simulink model "CryoDetXray"  (R2016b)
settings: Solver=ode45  StartTime=0.0  StopTime=10e-5  MaxStep=Tclk/4  RelTol=1e-3
values from neighbouring files (symbols this model uses):
  Fclk = Fadc    (= 307200000)    [setupCryoFPGAxray.m]
  Tclk = 1/Fclk    (= 3.25520833333e-09)    [setupCryoFPGAxray.m]
undefined symbols (not defined in the file or in its folder): AXI4, Lite, lpf, Naxi, xlipgetpartsetting
libraries: xbsIndex_r4 x1091, CryoDetLib x68, simulink x4, hdlsllib x1
(part 3 of 8)

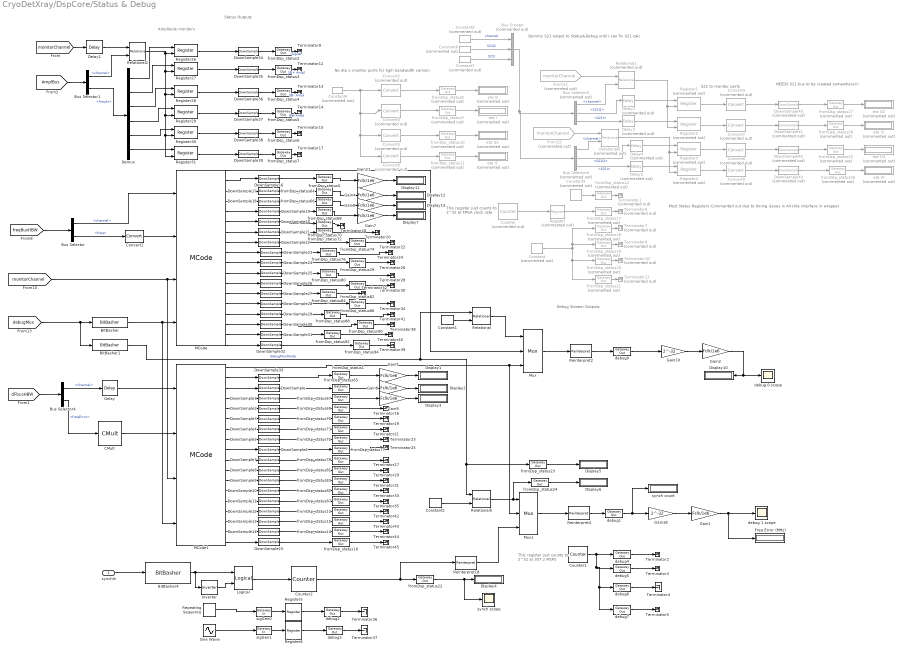
== system CryoDetXray/DspCore/Status & Debug ==
  note: Most Status Registers Commented out due to timing issues in AXI-lite interface in wrapper
  note: Dummy S21 output to Status&Debug until I can fix S21 calc
  note: No eta o monitor ports for hgih bandwidth version
  note: NEEDS S21 bus to be created somewhere!!!
  note: Amplitude monitors
  note: This register just counts to 2^32 at FPGA clock rate
  note: Status Outputs
  note: Debug Stream Outputs
  note: S21 to monitor ports
  note: This register just counts to 2^32 at 307.2 MSPS
  synchIn : Inport
  BitBasher : xbsIndex_r4/BitBasher  bitexpr=a={b[4:0]}  display_expr=on  sr_1=a  arith_type1=Unsigned  bin_pt1=0  sr_2=2  arith_type2=Unsigned  bin_pt2=0  sr_3=3  arith_type3=Unsigned  bin_pt3=0  sr_4=4  arith_type4=Unsigned  bin_pt4=0  dbl_ovrd=off  block_type=bitbasher
  BitBasher1 : xbsIndex_r4/BitBasher  bitexpr=a={b[6:5]}  display_expr=on  sr_1=a  arith_type1=Unsigned  bin_pt1=0  sr_2=2  arith_type2=Unsigned  bin_pt2=0  sr_3=3  arith_type3=Unsigned  bin_pt3=0  sr_4=4  arith_type4=Unsigned  bin_pt4=0  dbl_ovrd=off  block_type=bitbasher
  BitBasher4 : xbsIndex_r4/BitBasher  bitexpr=trig={Din[0]}  display_expr=on  sr_1=trig  arith_type1=Unsigned  bin_pt1=0  sr_2=2  arith_type2=Unsigned  bin_pt2=0  sr_3=3  arith_type3=Unsigned  bin_pt3=0  sr_4=4  arith_type4=Unsigned  bin_pt4=0  dbl_ovrd=off  block_type=bitbasher
  Bus Creator : BusCreator  Commented=on  Inputs=3
  Bus Selector : BusSelector  OutputSignals=channel,freq
  Bus Selector1 : BusSelector  OutputSignals=channel,Ampls
  Bus Selector4 : BusSelector  OutputSignals=channel,freqError
  Bus Selector5 : BusSelector  Commented=on  OutputSignals=channel,S21Q,S21I
  Bus Selector6 : BusSelector  Commented=on  OutputSignals=channel,S21Q,S21I
  CMult : xbsIndex_r4/CMult  const=16  gui_display_data_type=Fixed-point  const_n_bits=5  const_bin_pt=0  float_type=Single  exp_bits=8  fraction_bits=24  en=off  latency=3  precision=User Defined  arith_type="Signed  (2's comp)"  n_bits=32  bin_pt=31  quantization=Truncate  overflow=Saturate  use_behavioral_HDL=off  mem_type=Distributed RAM  pipeline=off  dbl_ovrd=off  block_type=cmult
  Constant : xbsIndex_r4/Constant  Commented=on  const=1.0  gui_display_data_type=Fixed-point  arith_type=Signed (2's comp)  n_bits=32  bin_pt=0  preci_type=Single  exp_width=8  frac_width=24  explicit_period=on  period=Tclk*Naxi  equ=P=C  opselect=C  inp2=PCIN>>17  opr=+  inp1=P  carry=CIN  dbl_ovrd=off  block_type=constant
  Constant1 : xbsIndex_r4/Constant  const=1  gui_display_data_type=Fixed-point  arith_type=Unsigned  n_bits=4  bin_pt=0  preci_type=Single  exp_width=8  frac_width=24  explicit_period=off  period=1  equ=P=C  opselect=C  inp2=PCIN>>17  opr=+  inp1=P  carry=CIN  dbl_ovrd=off  block_type=constant
  Constant2 : xbsIndex_r4/Constant  const=0  gui_display_data_type=Fixed-point  arith_type=Unsigned  n_bits=4  bin_pt=0  preci_type=Single  exp_width=8  frac_width=24  explicit_period=off  period=1  equ=P=C  opselect=C  inp2=PCIN>>17  opr=+  inp1=P  carry=CIN  dbl_ovrd=off  block_type=constant
  Constant3 : xbsIndex_r4/Constant  Commented=on  const=0  gui_display_data_type=Fixed-point  arith_type=Unsigned  n_bits=32  bin_pt=0  preci_type=Single  exp_width=8  frac_width=24  explicit_period=on  period=Tclk*Naxi  equ=P=C  opselect=C  inp2=PCIN>>17  opr=+  inp1=P  carry=CIN  dbl_ovrd=off  block_type=constant
  Constant4 : xbsIndex_r4/Constant  Commented=on  const=0  gui_display_data_type=Fixed-point  arith_type=Signed (2's comp)  n_bits=16  bin_pt=14  preci_type=Single  exp_width=8  frac_width=24  explicit_period=on  period=Tclk*Naxi  equ=P=C  opselect=C  inp2=PCIN>>17  opr=+  inp1=P  carry=CIN  dbl_ovrd=off  block_type=constant
  Constant5 : xbsIndex_r4/Constant  Commented=on  const=0  gui_display_data_type=Fixed-point  arith_type=Unsigned  n_bits=4  bin_pt=4  preci_type=Single  exp_width=8  frac_width=24  explicit_period=on  period=Tclk  equ=P=C  opselect=C  inp2=PCIN>>17  opr=+  inp1=P  carry=CIN  dbl_ovrd=off  block_type=constant
  Constant6 : xbsIndex_r4/Constant  Commented=on  const=0  gui_display_data_type=Fixed-point  arith_type=Signed (2's comp)  n_bits=32  bin_pt=14  preci_type=Single  exp_width=8  frac_width=24  explicit_period=on  period=Tclk  equ=P=C  opselect=C  inp2=PCIN>>17  opr=+  inp1=P  carry=CIN  dbl_ovrd=off  block_type=constant
  Constant7 : xbsIndex_r4/Constant  Commented=on  const=0  gui_display_data_type=Fixed-point  arith_type=Signed (2's comp)  n_bits=16  bin_pt=14  preci_type=Single  exp_width=8  frac_width=24  explicit_period=on  period=Tclk  equ=P=C  opselect=C  inp2=PCIN>>17  opr=+  inp1=P  carry=CIN  dbl_ovrd=off  block_type=constant
  Convert1 : xbsIndex_r4/Convert  gui_display_data_type=Fixed-point  arith_type="Signed  (2's comp)"  n_bits=32  bin_pt=31  float_type=Single  exp_bits=8  fraction_bits=24  quantization=Truncate  overflow=Wrap  en=off  latency=0  pipeline=off  dbl_ovrd=off  block_type=convert
  Convert{2..3,5..6} (4 alike) : xbsIndex_r4/Convert  Commented=on  gui_display_data_type=Fixed-point  arith_type="Signed  (2's comp)"  n_bits=32  bin_pt=14  float_type=Single  exp_bits=8  fraction_bits=24  quantization="Round  (unbiased: +/- Inf)"  overflow=Saturate  en=off  latency=1  pipeline=off  dbl_ovrd=off  block_type=convert
  Convert{4,7..9} (4 alike) : xbsIndex_r4/Convert  Commented=on  gui_display_data_type=Fixed-point  arith_type="Signed  (2's comp)"  n_bits=32  bin_pt=14  float_type=Single  exp_bits=8  fraction_bits=24  quantization="Round  (unbiased: +/- Inf)"  overflow=Saturate  en=off  latency=2  pipeline=off  dbl_ovrd=off  block_type=convert
  Counter : xbsIndex_r4/Counter  Commented=on  cnt_type=Free Running  cnt_to=Inf  operation=Up  start_count=0  cnt_by_val=1  arith_type=Unsigned  n_bits=32  bin_pt=0  load_pin=off  rst=off  en=off  explicit_period=on  period=Tclk*Naxi  use_behavioral_HDL=off  implementation=Fabric  dbl_ovrd=off  block_type=counter
  Counter1 : xbsIndex_r4/Counter  cnt_type=Free Running  cnt_to=Inf  operation=Up  start_count=0  cnt_by_val=1  arith_type=Unsigned  n_bits=32  bin_pt=0  load_pin=off  rst=off  en=off  explicit_period=on  period=Tclk  use_behavioral_HDL=off  implementation=Fabric  dbl_ovrd=off  block_type=counter
  Counter2 : xbsIndex_r4/Counter  cnt_type=Free Running  cnt_to=Inf  operation=Up  start_count=0  cnt_by_val=1  arith_type=Unsigned  n_bits=32  bin_pt=0  load_pin=off  rst=on  en=off  explicit_period=off  period=1  use_behavioral_HDL=on  implementation=Fabric  dbl_ovrd=off  block_type=counter
  Delay : xbsIndex_r4/Delay  rst=off  infoeditControl=Selection of Reset will increase slice count due to use of real FFs and instead of SRLs  en=off  latency=3  reg_retiming=off  dbl_ovrd=off  block_type=delay
      settings: infoedit=Hardware notes: A delay line is a chain, each link of which is an SRL16 or SRL32 followed by a flip-flop.
  Delay1 : xbsIndex_r4/Delay  rst=off  infoeditControl=Selection of Reset will increase slice count due to use of real FFs and instead of SRLs  en=off  latency=1  reg_retiming=on  dbl_ovrd=off  block_type=delay
  Delay{2..5} (4 alike) : xbsIndex_r4/Delay  Commented=on  rst=off  infoeditControl=Selection of Reset will increase slice count due to use of real FFs and instead of SRLs  en=off  latency=1  reg_retiming=on  dbl_ovrd=off  block_type=delay
  Demux : Demux  Outputs=6
  Display{1..7,10..13} (11 alike) : Display
      Display1 settings: Decimation=144
      Display10 settings: Decimation=144
      Display11 settings: Decimation=144
      Display12 settings: Decimation=144
      Display13 settings: Decimation=144
      Display2 settings: Decimation=144
      Display3 settings: Decimation=144
      Display7 settings: Decimation=144
  DownSample{,1..39} (40 alike) : CryoDetLib/DownSample
  DownSample{40..43} (4 alike) : CryoDetLib/DownSample  Commented=on
  Freq Error (MHz) : Display
      settings: Decimation=144
  From12 : From  Commented=on  GotoTag=monitorChannel  TagVisibility=global
  From15 : From  Commented=on  GotoTag=monitorChannel  TagVisibility=global
  Gain{1..2,4..9,21} (9 alike) : Gain  Gain=Fclk/1e6
  Gain10 : Gain  Gain=2^-32
  Gain18 : Gain  Gain=2^-32
  Inverter : xbsIndex_r4/Inverter  en=off  latency=1  dbl_ovrd=off  block_type=inv
  Logical : xbsIndex_r4/Logical  logical_function=AND  inputs=2  en=off  latency=1  precision=User Defined  arith_type=Boolean  n_bits=1  bin_pt=0  align_bp=on  dbl_ovrd=off  block_type=logical
  MCode : xbsIndex_r4/MCode  mfname=statusAndDebugPortsXray  explicit_period=off  period=1  inputsTable={'boundInpExpr'=>['','','',''],'inputs'=>['Chan','f','statusMux','debugMux']}  outputsTable={'outputs'=>['debugStream','fmon','f0','f1','f2','f3','f4','f5','f6','f7','f8','f9','f10','f11','f12','f13','f14','f15'],'suppressOut'=>['off','off','off','off','off','off','off','off','off','off','off','off','off','off','off','off','off','off']}  enable_stdout=off  enable_debug=off  suppress_output=on  defparams={}  hide_port_list={}  dbl_ovrd=off  block_type=mcode
  MCode1 : xbsIndex_r4/MCode  mfname=statusAndDebugPortsXray  explicit_period=off  period=1  inputsTable={'boundInpExpr'=>['','','',''],'inputs'=>['Chan','f','statusMux','debugMux']}  outputsTable={'outputs'=>['debugStream','fmon','f0','f1','f2','f3','f4','f5','f6','f7','f8','f9','f10','f11','f12','f13','f14','f15'],'suppressOut'=>['off','off','off','off','off','off','off','off','off','off','off','off','off','off','off','off','off','off']}  enable_stdout=off  enable_debug=on  suppress_output=on  defparams={}  hide_port_list={}  dbl_ovrd=off  block_type=mcode
  Mux : xbsIndex_r4/Mux  inputs=2  en=off  latency=0  precision=Full  arith_type=Unsigned  n_bits=16  bin_pt=14  quantization=Truncate  overflow=Wrap  dbl_ovrd=off  block_type=mux
  Mux1 : xbsIndex_r4/Mux  inputs=2  en=off  latency=0  precision=User Defined  arith_type="Signed  (2's comp)"  n_bits=32  bin_pt=31  quantization=Truncate  overflow=Saturate  dbl_ovrd=off  block_type=mux
  Register : xbsIndex_r4/Register  Commented=on  init=0  rst=off  en=off  dbl_ovrd=off  block_type=register
  Register{1..4} (4 alike) : xbsIndex_r4/Register  Commented=on  init=0  rst=off  en=on  dbl_ovrd=off  block_type=register
  Register{26..31} (6 alike) : xbsIndex_r4/Register  init=0  rst=off  en=on  dbl_ovrd=off  block_type=register
  Register5 : xbsIndex_r4/Register  init=1  rst=off  en=off  dbl_ovrd=off  block_type=register
  Register6 : xbsIndex_r4/Register  init=1  rst=off  en=off  dbl_ovrd=off  block_type=register
  Reinterpret18 : xbsIndex_r4/Reinterpret  force_arith_type=off  arith_type=Unsigned  force_bin_pt=on  bin_pt=32  block_type=reinterpret
  Reinterpret2 : xbsIndex_r4/Reinterpret  force_arith_type=on  arith_type=Unsigned  force_bin_pt=off  bin_pt=15  block_type=reinterpret
  Reinterpret4 : xbsIndex_r4/Reinterpret  force_arith_type=on  arith_type=Unsigned  force_bin_pt=off  bin_pt=15  block_type=reinterpret
  Relational : xbsIndex_r4/Relational  mode=a>b  op_type=Bool  en=off  latency=0  dbl_ovrd=off  block_type=relational
  Relational1 : xbsIndex_r4/Relational  Commented=on  mode=a=b  op_type=Bool  en=off  latency=1  dbl_ovrd=off  block_type=relational
  Relational2 : xbsIndex_r4/Relational  mode=a=b  op_type=Bool  en=off  latency=0  dbl_ovrd=off  block_type=relational
  Relational5 : xbsIndex_r4/Relational  mode=a!=b  op_type=Bool  en=off  latency=0  dbl_ovrd=off  block_type=relational
  Relational6 : xbsIndex_r4/Relational  Commented=on  mode=a=b  op_type=Bool  en=off  latency=1  dbl_ovrd=off  block_type=relational
  Repeating Sequence : simulink/Sources/Repeating Sequence  rep_seq_t="[0  2^32*Tclk]"  rep_seq_y=[0 1]
  Sine Wave : Sin  Amplitude=2^31  Bias=2^31  Frequency=2*pi*Fclk/2^32  SampleTime=0
  Terminator{1,6..8,10..11} (6 alike) : Terminator  Commented=on
  Terminator{2..5,9,12..45} (39 alike) : Terminator
  "debug 0 scope " : Scope
  debug 1 scope : Scope
  debug{0..7} (8 alike) : xbsIndex_r4/Gateway Out  inherit_from_input=on  hdl_port=on  rows=1  columns=1  UseAsDAC=off  DACChannel='1'  interface=None  automatic_assignment=on  address_offset=hex2dec('00')  intf_name=''  intf_description=''  timing_constraint=None  locs_specified=off  LOCs={}  io_standard={}  block_type=gatewayout
  eta I{,1..3} (4 alike) : Display  Commented=on
      settings: Decimation=144
  eta Q{,1..3} (4 alike) : Display  Commented=on
      settings: Decimation=144
  fromDsp_status0 : xbsIndex_r4/Gateway Out  inherit_from_input=on  hdl_port=on  rows=1  columns=1  UseAsDAC=off  DACChannel='1'  interface=AXI4-Lite  automatic_assignment=off  address_offset=hex2dec('00')  intf_name=''  intf_description=''  timing_constraint=None  locs_specified=off  LOCs={}  io_standard={}  block_type=gatewayout
  fromDsp_status1 : xbsIndex_r4/Gateway Out  inherit_from_input=on  hdl_port=on  rows=1  columns=1  UseAsDAC=off  DACChannel='1'  interface=AXI4-Lite  automatic_assignment=off  address_offset=hex2dec('04')  intf_name=''  intf_description=''  timing_constraint=None  locs_specified=off  LOCs={}  io_standard={}  block_type=gatewayout
  fromDsp_status10 : xbsIndex_r4/Gateway Out  Commented=on  inherit_from_input=on  hdl_port=on  rows=1  columns=1  UseAsDAC=off  DACChannel='1'  interface=AXI4-Lite  automatic_assignment=off  address_offset=hex2dec('28')  intf_name=''  intf_description=''  timing_constraint=None  locs_specified=off  LOCs={}  io_standard={}  block_type=gatewayout
  fromDsp_status11 : xbsIndex_r4/Gateway Out  Commented=on  inherit_from_input=on  hdl_port=on  rows=1  columns=1  UseAsDAC=off  DACChannel='1'  interface=AXI4-Lite  automatic_assignment=off  address_offset=hex2dec('2c')  intf_name=''  intf_description=''  timing_constraint=None  locs_specified=off  LOCs={}  io_standard={}  block_type=gatewayout
  fromDsp_status12 : xbsIndex_r4/Gateway Out  Commented=on  inherit_from_input=on  hdl_port=on  rows=1  columns=1  UseAsDAC=off  DACChannel='1'  interface=AXI4-Lite  automatic_assignment=off  address_offset=hex2dec('40')  intf_name=''  intf_description=''  timing_constraint=None  locs_specified=off  LOCs={}  io_standard={}  block_type=gatewayout
  fromDsp_status13 : xbsIndex_r4/Gateway Out  inherit_from_input=on  hdl_port=on  rows=1  columns=1  UseAsDAC=off  DACChannel='1'  interface=AXI4-Lite  automatic_assignment=off  address_offset=hex2dec('164')  intf_name=''  intf_description=''  timing_constraint=None  locs_specified=off  LOCs={}  io_standard={}  block_type=gatewayout
  fromDsp_status14 : xbsIndex_r4/Gateway Out  inherit_from_input=on  hdl_port=on  rows=1  columns=1  UseAsDAC=off  DACChannel='1'  interface=AXI4-Lite  automatic_assignment=off  address_offset=hex2dec('174')  intf_name=''  intf_description=''  timing_constraint=None  locs_specified=off  LOCs={}  io_standard={}  block_type=gatewayout
  fromDsp_status15 : xbsIndex_r4/Gateway Out  inherit_from_input=on  hdl_port=on  rows=1  columns=1  UseAsDAC=off  DACChannel='1'  interface=AXI4-Lite  automatic_assignment=off  address_offset=hex2dec('16c')  intf_name=''  intf_description=''  timing_constraint=None  locs_specified=off  LOCs={}  io_standard={}  block_type=gatewayout
  fromDsp_status16 : xbsIndex_r4/Gateway Out  inherit_from_input=on  hdl_port=on  rows=1  columns=1  UseAsDAC=off  DACChannel='1'  interface=AXI4-Lite  automatic_assignment=off  address_offset=hex2dec('17c')  intf_name=''  intf_description=''  timing_constraint=None  locs_specified=off  LOCs={}  io_standard={}  block_type=gatewayout
  fromDsp_status17 : xbsIndex_r4/Gateway Out  Commented=on  inherit_from_input=on  hdl_port=on  rows=1  columns=1  UseAsDAC=off  DACChannel='1'  interface=AXI4-Lite  automatic_assignment=off  address_offset=hex2dec('44')  intf_name=''  intf_description=''  timing_constraint=None  locs_specified=off  LOCs={}  io_standard={}  block_type=gatewayout
  fromDsp_status18 : xbsIndex_r4/Gateway Out  Commented=on  inherit_from_input=on  hdl_port=on  rows=1  columns=1  UseAsDAC=off  DACChannel='1'  interface=AXI4-Lite  automatic_assignment=off  address_offset=hex2dec('48')  intf_name=''  intf_description=''  timing_constraint=None  locs_specified=off  LOCs={}  io_standard={}  block_type=gatewayout
  fromDsp_status19 : xbsIndex_r4/Gateway Out  Commented=on  inherit_from_input=on  hdl_port=on  rows=1  columns=1  UseAsDAC=off  DACChannel='1'  interface=AXI4-Lite  automatic_assignment=off  address_offset=hex2dec('4c')  intf_name=''  intf_description=''  timing_constraint=None  locs_specified=off  LOCs={}  io_standard={}  block_type=gatewayout
  fromDsp_status2 : xbsIndex_r4/Gateway Out  inherit_from_input=on  hdl_port=on  rows=1  columns=1  UseAsDAC=off  DACChannel='1'  interface=AXI4-Lite  automatic_assignment=off  address_offset=hex2dec('08')  intf_name=''  intf_description=''  timing_constraint=None  locs_specified=off  LOCs={}  io_standard={}  block_type=gatewayout
  fromDsp_status20 : xbsIndex_r4/Gateway Out  Commented=on  inherit_from_input=on  hdl_port=on  rows=1  columns=1  UseAsDAC=off  DACChannel='1'  interface=AXI4-Lite  automatic_assignment=off  address_offset=hex2dec('50')  intf_name=''  intf_description=''  timing_constraint=None  locs_specified=off  LOCs={}  io_standard={}  block_type=gatewayout
  fromDsp_status21 : xbsIndex_r4/Gateway Out  Commented=on  inherit_from_input=on  hdl_port=on  rows=1  columns=1  UseAsDAC=off  DACChannel='1'  interface=AXI4-Lite  automatic_assignment=off  address_offset=hex2dec('54')  intf_name=''  intf_description=''  timing_constraint=None  locs_specified=off  LOCs={}  io_standard={}  block_type=gatewayout
  fromDsp_status22 : xbsIndex_r4/Gateway Out  inherit_from_input=on  hdl_port=off  rows=1  columns=1  UseAsDAC=off  DACChannel='1'  interface=AXI4-Lite  automatic_assignment=off  address_offset=hex2dec('30')  intf_name=''  intf_description=''  timing_constraint=None  locs_specified=off  LOCs={}  io_standard={}  block_type=gatewayout
  fromDsp_status23 : xbsIndex_r4/Gateway Out  inherit_from_input=on  hdl_port=off  rows=1  columns=1  UseAsDAC=off  DACChannel='1'  interface=AXI4-Lite  automatic_assignment=off  address_offset=hex2dec('30')  intf_name=''  intf_description=''  timing_constraint=None  locs_specified=off  LOCs={}  io_standard={}  block_type=gatewayout
  fromDsp_status24 : xbsIndex_r4/Gateway Out  inherit_from_input=on  hdl_port=off  rows=1  columns=1  UseAsDAC=off  DACChannel='1'  interface=AXI4-Lite  automatic_assignment=off  address_offset=hex2dec('30')  intf_name=''  intf_description=''  timing_constraint=None  locs_specified=off  LOCs={}  io_standard={}  block_type=gatewayout
  fromDsp_status25 : xbsIndex_r4/Gateway Out  Commented=on  inherit_from_input=on  hdl_port=on  rows=1  columns=1  UseAsDAC=off  DACChannel='1'  interface=AXI4-Lite  automatic_assignment=off  address_offset=hex2dec('38')  intf_name=''  intf_description=''  timing_constraint=None  locs_specified=off  LOCs={}  io_standard={}  block_type=gatewayout
  fromDsp_status26 : xbsIndex_r4/Gateway Out  Commented=on  inherit_from_input=on  hdl_port=on  rows=1  columns=1  UseAsDAC=off  DACChannel='1'  interface=AXI4-Lite  automatic_assignment=off  address_offset=hex2dec('3c')  intf_name=''  intf_description=''  timing_constraint=None  locs_specified=off  LOCs={}  io_standard={}  block_type=gatewayout
  fromDsp_status27 : xbsIndex_r4/Gateway Out  Commented=on  inherit_from_input=on  hdl_port=on  rows=1  columns=1  UseAsDAC=off  DACChannel='1'  interface=AXI4-Lite  automatic_assignment=off  address_offset=hex2dec('30')  intf_name=''  intf_description=''  timing_constraint=None  locs_specified=off  LOCs={}  io_standard={}  block_type=gatewayout
  fromDsp_status28 : xbsIndex_r4/Gateway Out  Commented=on  inherit_from_input=on  hdl_port=on  rows=1  columns=1  UseAsDAC=off  DACChannel='1'  interface=AXI4-Lite  automatic_assignment=off  address_offset=hex2dec('34')  intf_name=''  intf_description=''  timing_constraint=None  locs_specified=off  LOCs={}  io_standard={}  block_type=gatewayout
  fromDsp_status29 : xbsIndex_r4/Gateway Out  inherit_from_input=on  hdl_port=on  rows=1  columns=1  UseAsDAC=off  DACChannel='1'  interface=AXI4-Lite  automatic_assignment=off  address_offset=hex2dec('138')  intf_name=''  intf_description=''  timing_constraint=None  locs_specified=off  LOCs={}  io_standard={}  block_type=gatewayout
  fromDsp_status3 : xbsIndex_r4/Gateway Out  inherit_from_input=on  hdl_port=on  rows=1  columns=1  UseAsDAC=off  DACChannel='1'  interface=AXI4-Lite  automatic_assignment=off  address_offset=hex2dec('0C')  intf_name=''  intf_description=''  timing_constraint=None  locs_specified=off  LOCs={}  io_standard={}  block_type=gatewayout
  fromDsp_status4 : xbsIndex_r4/Gateway Out  inherit_from_input=on  hdl_port=on  rows=1  columns=1  UseAsDAC=off  DACChannel='1'  interface=AXI4-Lite  automatic_assignment=off  address_offset=hex2dec('10')  intf_name=''  intf_description=''  timing_constraint=None  locs_specified=off  LOCs={}  io_standard={}  block_type=gatewayout
  fromDsp_status5 : xbsIndex_r4/Gateway Out  inherit_from_input=on  hdl_port=on  rows=1  columns=1  UseAsDAC=off  DACChannel='1'  interface=AXI4-Lite  automatic_assignment=off  address_offset=hex2dec('14')  intf_name=''  intf_description=''  timing_constraint=None  locs_specified=off  LOCs={}  io_standard={}  block_type=gatewayout
  fromDsp_status6 : xbsIndex_r4/Gateway Out  inherit_from_input=on  hdl_port=on  rows=1  columns=1  UseAsDAC=off  DACChannel='1'  interface=AXI4-Lite  automatic_assignment=off  address_offset=hex2dec('18')  intf_name=''  intf_description=''  timing_constraint=None  locs_specified=off  LOCs={}  io_standard={}  block_type=gatewayout
  fromDsp_status64 : xbsIndex_r4/Gateway Out  inherit_from_input=on  hdl_port=on  rows=1  columns=1  UseAsDAC=off  DACChannel='1'  interface=AXI4-Lite  automatic_assignment=off  address_offset=hex2dec('100')  intf_name=''  intf_description=''  timing_constraint=None  locs_specified=off  LOCs={}  io_standard={}  block_type=gatewayout
  fromDsp_status65 : xbsIndex_r4/Gateway Out  inherit_from_input=on  hdl_port=on  rows=1  columns=1  UseAsDAC=off  DACChannel='1'  interface=AXI4-Lite  automatic_assignment=off  address_offset=hex2dec('104')  intf_name=''  intf_description=''  timing_constraint=None  locs_specified=off  LOCs={}  io_standard={}  block_type=gatewayout
  fromDsp_status66 : xbsIndex_r4/Gateway Out  inherit_from_input=on  hdl_port=on  rows=1  columns=1  UseAsDAC=off  DACChannel='1'  interface=AXI4-Lite  automatic_assignment=off  address_offset=hex2dec('108')  intf_name=''  intf_description=''  timing_constraint=None  locs_specified=off  LOCs={}  io_standard={}  block_type=gatewayout
  fromDsp_status67 : xbsIndex_r4/Gateway Out  inherit_from_input=on  hdl_port=on  rows=1  columns=1  UseAsDAC=off  DACChannel='1'  interface=AXI4-Lite  automatic_assignment=off  address_offset=hex2dec('10c')  intf_name=''  intf_description=''  timing_constraint=None  locs_specified=off  LOCs={}  io_standard={}  block_type=gatewayout
  fromDsp_status68 : xbsIndex_r4/Gateway Out  inherit_from_input=on  hdl_port=on  rows=1  columns=1  UseAsDAC=off  DACChannel='1'  interface=AXI4-Lite  automatic_assignment=off  address_offset=hex2dec('110')  intf_name=''  intf_description=''  timing_constraint=None  locs_specified=off  LOCs={}  io_standard={}  block_type=gatewayout
  fromDsp_status69 : xbsIndex_r4/Gateway Out  inherit_from_input=on  hdl_port=on  rows=1  columns=1  UseAsDAC=off  DACChannel='1'  interface=AXI4-Lite  automatic_assignment=off  address_offset=hex2dec('114')  intf_name=''  intf_description=''  timing_constraint=None  locs_specified=off  LOCs={}  io_standard={}  block_type=gatewayout
  fromDsp_status7 : xbsIndex_r4/Gateway Out  inherit_from_input=on  hdl_port=on  rows=1  columns=1  UseAsDAC=off  DACChannel='1'  interface=AXI4-Lite  automatic_assignment=off  address_offset=hex2dec('1C')  intf_name=''  intf_description=''  timing_constraint=None  locs_specified=off  LOCs={}  io_standard={}  block_type=gatewayout
  fromDsp_status70 : xbsIndex_r4/Gateway Out  inherit_from_input=on  hdl_port=on  rows=1  columns=1  UseAsDAC=off  DACChannel='1'  interface=AXI4-Lite  automatic_assignment=off  address_offset=hex2dec('118')  intf_name=''  intf_description=''  timing_constraint=None  locs_specified=off  LOCs={}  io_standard={}  block_type=gatewayout
  fromDsp_status71 : xbsIndex_r4/Gateway Out  inherit_from_input=on  hdl_port=on  rows=1  columns=1  UseAsDAC=off  DACChannel='1'  interface=AXI4-Lite  automatic_assignment=off  address_offset=hex2dec('11c')  intf_name=''  intf_description=''  timing_constraint=None  locs_specified=off  LOCs={}  io_standard={}  block_type=gatewayout
  fromDsp_status72 : xbsIndex_r4/Gateway Out  inherit_from_input=on  hdl_port=on  rows=1  columns=1  UseAsDAC=off  DACChannel='1'  interface=AXI4-Lite  automatic_assignment=off  address_offset=hex2dec('120')  intf_name=''  intf_description=''  timing_constraint=None  locs_specified=off  LOCs={}  io_standard={}  block_type=gatewayout
  fromDsp_status73 : xbsIndex_r4/Gateway Out  inherit_from_input=on  hdl_port=on  rows=1  columns=1  UseAsDAC=off  DACChannel='1'  interface=AXI4-Lite  automatic_assignment=off  address_offset=hex2dec('124')  intf_name=''  intf_description=''  timing_constraint=None  locs_specified=off  LOCs={}  io_standard={}  block_type=gatewayout
  fromDsp_status74 : xbsIndex_r4/Gateway Out  inherit_from_input=on  hdl_port=on  rows=1  columns=1  UseAsDAC=off  DACChannel='1'  interface=AXI4-Lite  automatic_assignment=off  address_offset=hex2dec('128')  intf_name=''  intf_description=''  timing_constraint=None  locs_specified=off  LOCs={}  io_standard={}  block_type=gatewayout
  fromDsp_status75 : xbsIndex_r4/Gateway Out  inherit_from_input=on  hdl_port=on  rows=1  columns=1  UseAsDAC=off  DACChannel='1'  interface=AXI4-Lite  automatic_assignment=off  address_offset=hex2dec('12c')  intf_name=''  intf_description=''  timing_constraint=None  locs_specified=off  LOCs={}  io_standard={}  block_type=gatewayout
  fromDsp_status76 : xbsIndex_r4/Gateway Out  inherit_from_input=on  hdl_port=on  rows=1  columns=1  UseAsDAC=off  DACChannel='1'  interface=AXI4-Lite  automatic_assignment=off  address_offset=hex2dec('130')  intf_name=''  intf_description=''  timing_constraint=None  locs_specified=off  LOCs={}  io_standard={}  block_type=gatewayout
  fromDsp_status77 : xbsIndex_r4/Gateway Out  inherit_from_input=on  hdl_port=on  rows=1  columns=1  UseAsDAC=off  DACChannel='1'  interface=AXI4-Lite  automatic_assignment=off  address_offset=hex2dec('134')  intf_name=''  intf_description=''  timing_constraint=None  locs_specified=off  LOCs={}  io_standard={}  block_type=gatewayout
  fromDsp_status79 : xbsIndex_r4/Gateway Out  inherit_from_input=on  hdl_port=on  rows=1  columns=1  UseAsDAC=off  DACChannel='1'  interface=AXI4-Lite  automatic_assignment=off  address_offset=hex2dec('13c')  intf_name=''  intf_description=''  timing_constraint=None  locs_specified=off  LOCs={}  io_standard={}  block_type=gatewayout
  fromDsp_status8 : xbsIndex_r4/Gateway Out  Commented=on  inherit_from_input=on  hdl_port=on  rows=1  columns=1  UseAsDAC=off  DACChannel='1'  interface=AXI4-Lite  automatic_assignment=off  address_offset=hex2dec('20')  intf_name=''  intf_description=''  timing_constraint=None  locs_specified=off  LOCs={}  io_standard={}  block_type=gatewayout
  fromDsp_status80 : xbsIndex_r4/Gateway Out  inherit_from_input=on  hdl_port=on  rows=1  columns=1  UseAsDAC=off  DACChannel='1'  interface=AXI4-Lite  automatic_assignment=off  address_offset=hex2dec('140')  intf_name=''  intf_description=''  timing_constraint=None  locs_specified=off  LOCs={}  io_standard={}  block_type=gatewayout
  fromDsp_status81 : xbsIndex_r4/Gateway Out  inherit_from_input=on  hdl_port=on  rows=1  columns=1  UseAsDAC=off  DACChannel='1'  interface=AXI4-Lite  automatic_assignment=off  address_offset=hex2dec('144')  intf_name=''  intf_description=''  timing_constraint=None  locs_specified=off  LOCs={}  io_standard={}  block_type=gatewayout
  fromDsp_status82 : xbsIndex_r4/Gateway Out  inherit_from_input=on  hdl_port=on  rows=1  columns=1  UseAsDAC=off  DACChannel='1'  interface=AXI4-Lite  automatic_assignment=off  address_offset=hex2dec('148')  intf_name=''  intf_description=''  timing_constraint=None  locs_specified=off  LOCs={}  io_standard={}  block_type=gatewayout
  fromDsp_status83 : xbsIndex_r4/Gateway Out  inherit_from_input=on  hdl_port=on  rows=1  columns=1  UseAsDAC=off  DACChannel='1'  interface=AXI4-Lite  automatic_assignment=off  address_offset=hex2dec('14c')  intf_name=''  intf_description=''  timing_constraint=None  locs_specified=off  LOCs={}  io_standard={}  block_type=gatewayout
  fromDsp_status84 : xbsIndex_r4/Gateway Out  inherit_from_input=on  hdl_port=on  rows=1  columns=1  UseAsDAC=off  DACChannel='1'  interface=AXI4-Lite  automatic_assignment=off  address_offset=hex2dec('150')  intf_name=''  intf_description=''  timing_constraint=None  locs_specified=off  LOCs={}  io_standard={}  block_type=gatewayout
  fromDsp_status85 : xbsIndex_r4/Gateway Out  inherit_from_input=on  hdl_port=on  rows=1  columns=1  UseAsDAC=off  DACChannel='1'  interface=AXI4-Lite  automatic_assignment=off  address_offset=hex2dec('154')  intf_name=''  intf_description=''  timing_constraint=None  locs_specified=off  LOCs={}  io_standard={}  block_type=gatewayout
  fromDsp_status86 : xbsIndex_r4/Gateway Out  inherit_from_input=on  hdl_port=on  rows=1  columns=1  UseAsDAC=off  DACChannel='1'  interface=AXI4-Lite  automatic_assignment=off  address_offset=hex2dec('158')  intf_name=''  intf_description=''  timing_constraint=None  locs_specified=off  LOCs={}  io_standard={}  block_type=gatewayout
  fromDsp_status87 : xbsIndex_r4/Gateway Out  inherit_from_input=on  hdl_port=on  rows=1  columns=1  UseAsDAC=off  DACChannel='1'  interface=AXI4-Lite  automatic_assignment=off  address_offset=hex2dec('15c')  intf_name=''  intf_description=''  timing_constraint=None  locs_specified=off  LOCs={}  io_standard={}  block_type=gatewayout
  fromDsp_status88 : xbsIndex_r4/Gateway Out  inherit_from_input=on  hdl_port=on  rows=1  columns=1  UseAsDAC=off  DACChannel='1'  interface=AXI4-Lite  automatic_assignment=off  address_offset=hex2dec('160')  intf_name=''  intf_description=''  timing_constraint=None  locs_specified=off  LOCs={}  io_standard={}  block_type=gatewayout
  fromDsp_status9 : xbsIndex_r4/Gateway Out  Commented=on  inherit_from_input=on  hdl_port=on  rows=1  columns=1  UseAsDAC=off  DACChannel='1'  interface=AXI4-Lite  automatic_assignment=off  address_offset=hex2dec('24')  intf_name=''  intf_description=''  timing_constraint=None  locs_specified=off  LOCs={}  io_standard={}  block_type=gatewayout
  fromDsp_status90 : xbsIndex_r4/Gateway Out  inherit_from_input=on  hdl_port=on  rows=1  columns=1  UseAsDAC=off  DACChannel='1'  interface=AXI4-Lite  automatic_assignment=off  address_offset=hex2dec('168')  intf_name=''  intf_description=''  timing_constraint=None  locs_specified=off  LOCs={}  io_standard={}  block_type=gatewayout
  fromDsp_status92 : xbsIndex_r4/Gateway Out  inherit_from_input=on  hdl_port=on  rows=1  columns=1  UseAsDAC=off  DACChannel='1'  interface=AXI4-Lite  automatic_assignment=off  address_offset=hex2dec('170')  intf_name=''  intf_description=''  timing_constraint=None  locs_specified=off  LOCs={}  io_standard={}  block_type=gatewayout
  fromDsp_status94 : xbsIndex_r4/Gateway Out  inherit_from_input=on  hdl_port=on  rows=1  columns=1  UseAsDAC=off  DACChannel='1'  interface=AXI4-Lite  automatic_assignment=off  address_offset=hex2dec('178')  intf_name=''  intf_description=''  timing_constraint=None  locs_specified=off  LOCs={}  io_standard={}  block_type=gatewayout
  sigGen0 : xbsIndex_r4/Gateway In  gui_display_data_type=Fixed-point  arith_type=Unsigned  n_bits=32  bin_pt=0  preci_type=Single  exp_width=8  frac_width=24  rows=1  columns=1  quantization=Truncate  overflow=Wrap  period=Ts  UseAsADC=off  ADCChannel='1'  interface=None  automatic_assignment=on  address_offset=hex2dec('00')  intf_name=''  intf_description=''  default_value=0  timing_constraint=None  locs_specified=off  LOCs={}  io_standard={}  inherit_from_input=off  hdl_port=on  dbl_ovrd=off  block_type=gatewayin
  sigGen1 : xbsIndex_r4/Gateway In  gui_display_data_type=Fixed-point  arith_type=Unsigned  n_bits=32  bin_pt=0  preci_type=Single  exp_width=8  frac_width=24  rows=1  columns=1  quantization=Truncate  overflow=Wrap  period=Ts  UseAsADC=off  ADCChannel='1'  interface=None  automatic_assignment=on  address_offset=hex2dec('00')  intf_name=''  intf_description=''  default_value=0  timing_constraint=None  locs_specified=off  LOCs={}  io_standard={}  inherit_from_input=off  hdl_port=on  dbl_ovrd=off  block_type=gatewayin
  synch count : Display
  synch scope : Scope
  wires:
  debug0/1 -> Gain10/1
  [monitorChannel] -> Delay1/1
  Reinterpret2/1 -> debug0/1
  Mux/1 -> Reinterpret2/1
  Gain2/1 -> Display10/1, "debug 0 scope "/1
  Gain10/1 -> Gain2/1
  [AmplBus] -> Bus Selector1/1
  Bus Selector1/1 -> Relational2/2  "<channel>"
  Relational2/1 -> Register27/2, Register28/2, Register29/2, Register30/2, Register31/2, Register26/2
  Demux/6 -> Register31/1
  Demux/5 -> Register30/1
  Demux/4 -> Register29/1
  Demux/3 -> Register28/1
  Demux/2 -> Register27/1
  Demux/1 -> Register26/1
  Bus Selector1/2 -> Demux/1  "<Ampls>"
  fromDsp_status8/1 -> eta Q/1
  fromDsp_status9/1 -> eta I/1
  Convert2/1 -> fromDsp_status8/1
  Convert3/1 -> fromDsp_status9/1
  fromDsp_status10/1 -> eta Q1/1
  fromDsp_status11/1 -> eta I1/1
  Convert5/1 -> fromDsp_status10/1
  Convert6/1 -> fromDsp_status11/1
  Constant/1 -> fromDsp_status21/1, fromDsp_status20/1, fromDsp_status18/1, fromDsp_status19/1
  Reinterpret4/1 -> debug1/1
  Mux1/1 -> Reinterpret4/1
  Gain18/1 -> Gain1/1
  Gain1/1 -> Freq Error (MHz)/1, debug 1 scope/1
  [freqBusHBW] -> Bus Selector/1
  Bus Selector/1 -> MCode/1  "<channel>"
  Bus Selector/2 -> Convert1/1  "<freq>"
  Convert1/1 -> MCode/2
  [monitorChannel] -> MCode/3, MCode1/3
  [debugMux] -> BitBasher1/1, BitBasher/1
  [dFbusHBW] -> Bus Selector4/1
  Bus Selector4/1 -> Delay/1  "<channel>"
  Bus Selector4/2 -> CMult/1  "<freqError>"
  Gain21/1 -> Display11/1
  Gain4/1 -> Display12/1
  Gain6/1 -> Display13/1
  fromDsp_status0/1 -> Gain21/1
  fromDsp_status64/1 -> Gain4/1
  fromDsp_status66/1 -> Gain6/1
  CMult/1 -> MCode1/2
  BitBasher/1 -> MCode/4, MCode1/4
  MCode/1 -> Mux/2
  MCode1/1 -> Mux1/2, Mux/3
  BitBasher1/1 -> Relational/1, Relational5/1, fromDsp_status23/1  "debugMuxMode"
  Relational/1 -> Mux/1
  Constant1/1 -> Relational/2
  Constant2/1 -> Relational5/2
  Relational5/1 -> fromDsp_status24/1, Mux1/1
  Gain5/1 -> Display1/1
  Gain8/1 -> Display2/1
  Gain9/1 -> Display3/1
  fromDsp_status1/1 -> Gain5/1
  fromDsp_status65/1 -> Gain8/1
  fromDsp_status67/1 -> Gain9/1
  MCode1/7 -> DownSample4/1
  MCode1/12 -> DownSample9/1
  MCode1/10 -> DownSample7/1
  MCode1/9 -> DownSample6/1
  MCode1/8 -> DownSample5/1
  Counter2/1 -> Reinterpret18/1, fromDsp_status22/1
  fromDsp_status22/1 -> synch scope/1, Display4/1
  fromDsp_status23/1 -> Display5/1
  fromDsp_status24/1 -> Display6/1
  Reinterpret18/1 -> Mux1/3
  debug1/1 -> synch count/1, Gain18/1
  Gain7/1 -> Display7/1
  fromDsp_status68/1 -> Gain7/1
  fromDsp_status17/1 -> Terminator6/1
  fromDsp_status18/1 -> Terminator7/1
  fromDsp_status19/1 -> Terminator8/1
  fromDsp_status2/1 -> Terminator9/1  "Signal"
  fromDsp_status20/1 -> Terminator10/1
  fromDsp_status21/1 -> Terminator11/1
  fromDsp_status3/1 -> Terminator12/1  "SB+ Ampl"
  fromDsp_status4/1 -> Terminator13/1  "SB- Ampl"
  fromDsp_status5/1 -> Terminator14/1  "Ref Ampl"
  fromDsp_status6/1 -> Terminator15/1
  fromDsp_status69/1 -> Terminator16/1
  fromDsp_status7/1 -> Terminator17/1
  fromDsp_status70/1 -> Terminator18/1
  fromDsp_status71/1 -> Terminator19/1
  fromDsp_status72/1 -> Terminator20/1
  fromDsp_status73/1 -> Terminator21/1
  fromDsp_status74/1 -> Terminator22/1
  fromDsp_status75/1 -> Terminator23/1
  fromDsp_status76/1 -> Terminator24/1
  fromDsp_status77/1 -> Terminator25/1
  fromDsp_status29/1 -> Terminator26/1
  fromDsp_status79/1 -> Terminator27/1
  fromDsp_status81/1 -> Terminator29/1
  fromDsp_status83/1 -> Terminator31/1
  fromDsp_status84/1 -> Terminator32/1
  fromDsp_status86/1 -> Terminator34/1
  fromDsp_status87/1 -> Terminator35/1
  Delay/1 -> MCode1/1
  Register1/1 -> Convert4/1
  Register2/1 -> Convert7/1
  Bus Selector5/1 -> Relational1/2  "<channel>"
  Bus Selector5/2 -> Delay2/1  "<S21Q>"
  Bus Selector5/3 -> Delay3/1  "<S21I>"
  Relational1/1 -> Register2/2, Register1/2
  fromDsp_status27/1 -> eta Q2/1
  fromDsp_status28/1 -> eta I2/1
  Register3/1 -> Convert8/1
  Register4/1 -> Convert9/1
  Bus Selector6/1 -> Relational6/2  "<channel>"
  Bus Selector6/2 -> Delay4/1  "<S21Q>"
  Bus Selector6/3 -> Delay5/1  "<S21I>"
  Relational6/1 -> Register4/2, Register3/2
  fromDsp_status25/1 -> eta Q3/1
  fromDsp_status26/1 -> eta I3/1
  Bus Creator/1 -> Bus Selector6/1, Bus Selector5/1
  From15/1 -> Relational6/1
  From12/1 -> Relational1/1
  Counter/1 -> Register/1
  Counter1/1 -> debug6/1, debug7/1, debug5/1, debug4/1
  debug4/1 -> Terminator2/1
  debug5/1 -> Terminator3/1
  fromDsp_status12/1 -> Terminator1/1
  Constant3/1 -> fromDsp_status12/1
  synchIn/1 -> BitBasher4/1
  BitBasher4/1 -> Inverter/1, Logical/1
  Inverter/1 -> Logical/2
  Logical/1 -> Counter2/1
  Constant4/1 -> Convert3/1, Convert5/1, Convert6/1, Convert2/1
  Delay1/1 -> Relational2/1
  Delay2/1 -> Register1/1
  Delay3/1 -> Register2/1
  Delay4/1 -> Register3/1
  Delay5/1 -> Register4/1
  debug6/1 -> Terminator4/1
  debug7/1 -> Terminator5/1
  sigGen0/1 -> Register5/1
  Register5/1 -> debug2/1
  sigGen1/1 -> Register6/1
  Register6/1 -> debug3/1
  debug2/1 -> Terminator36/1
  debug3/1 -> Terminator37/1
  Repeating Sequence/1 -> sigGen0/1
  Sine Wave/1 -> sigGen1/1
  Constant7/1 -> Bus Creator/3  "S21I"
  Constant6/1 -> Bus Creator/2  "S21Q"
  Constant5/1 -> Bus Creator/1  "channel"
  Register26/1 -> DownSample34/1
  Register27/1 -> DownSample35/1
  Register28/1 -> DownSample36/1
  Register29/1 -> DownSample37/1
  Register30/1 -> DownSample38/1
  Register31/1 -> DownSample39/1
  fromDsp_status82/1 -> Terminator30/1
  fromDsp_status80/1 -> Terminator28/1
  MCode/2 -> DownSample16/1
  MCode/3 -> DownSample17/1
  MCode/4 -> DownSample18/1
  MCode/5 -> DownSample19/1
  MCode/6 -> DownSample20/1
  MCode/7 -> DownSample21/1
  MCode/8 -> DownSample22/1
  MCode/9 -> DownSample23/1
  MCode/10 -> DownSample24/1
  MCode/11 -> DownSample25/1
  MCode/12 -> DownSample26/1
  MCode/14 -> DownSample28/1
  MCode/13 -> DownSample27/1
  MCode/15 -> DownSample29/1
  MCode/16 -> DownSample30/1
  MCode/17 -> DownSample31/1
  MCode/18 -> DownSample32/1
  fromDsp_status90/1 -> Terminator38/1
  fromDsp_status94/1 -> Terminator39/1
  fromDsp_status92/1 -> Terminator40/1
  fromDsp_status88/1 -> Terminator41/1
  MCode1/3 -> DownSample/1
  MCode1/4 -> DownSample1/1
  MCode1/6 -> DownSample3/1
  DownSample4/1 -> fromDsp_status73/1
  DownSample5/1 -> fromDsp_status75/1
  DownSample6/1 -> fromDsp_status77/1
  MCode1/11 -> DownSample8/1
  MCode1/13 -> DownSample10/1
  MCode1/14 -> DownSample11/1
  MCode1/15 -> DownSample12/1
  MCode1/16 -> DownSample13/1
  MCode1/17 -> DownSample14/1
  MCode1/18 -> DownSample15/1
  Convert9/1 -> DownSample43/1
  Convert8/1 -> DownSample42/1
  Convert7/1 -> DownSample41/1
  Convert4/1 -> DownSample40/1
  MCode1/2 -> DownSample33/1
  DownSample/1 -> fromDsp_status65/1
  DownSample1/1 -> fromDsp_status67/1
  MCode1/5 -> DownSample2/1
  DownSample2/1 -> fromDsp_status69/1
  DownSample3/1 -> fromDsp_status71/1
  DownSample7/1 -> fromDsp_status79/1
  DownSample8/1 -> fromDsp_status81/1
  DownSample9/1 -> fromDsp_status83/1
  DownSample10/1 -> fromDsp_status85/1
  DownSample11/1 -> fromDsp_status87/1
  DownSample12/1 -> fromDsp_status13/1
  DownSample13/1 -> fromDsp_status15/1
  DownSample14/1 -> fromDsp_status14/1
  DownSample15/1 -> fromDsp_status16/1
  DownSample16/1 -> fromDsp_status0/1
  DownSample17/1 -> fromDsp_status64/1
  DownSample18/1 -> fromDsp_status66/1
  DownSample19/1 -> fromDsp_status68/1
  DownSample20/1 -> fromDsp_status70/1
  DownSample21/1 -> fromDsp_status72/1
  DownSample22/1 -> fromDsp_status74/1
  DownSample23/1 -> fromDsp_status76/1
  DownSample24/1 -> fromDsp_status29/1
  DownSample25/1 -> fromDsp_status80/1
  DownSample26/1 -> fromDsp_status82/1
  DownSample27/1 -> fromDsp_status84/1
  DownSample28/1 -> fromDsp_status86/1
  DownSample29/1 -> fromDsp_status88/1
  DownSample30/1 -> fromDsp_status90/1
  DownSample31/1 -> fromDsp_status92/1
  DownSample32/1 -> fromDsp_status94/1
  DownSample33/1 -> fromDsp_status1/1
  DownSample34/1 -> fromDsp_status2/1
  DownSample35/1 -> fromDsp_status3/1
  DownSample36/1 -> fromDsp_status4/1
  DownSample37/1 -> fromDsp_status5/1
  DownSample38/1 -> fromDsp_status6/1
  DownSample39/1 -> fromDsp_status7/1
  Register/1 -> fromDsp_status17/1
  DownSample40/1 -> fromDsp_status27/1
  DownSample41/1 -> fromDsp_status28/1
  DownSample42/1 -> fromDsp_status25/1
  DownSample43/1 -> fromDsp_status26/1
  fromDsp_status85/1 -> Terminator33/1
  fromDsp_status13/1 -> Terminator42/1
  fromDsp_status15/1 -> Terminator43/1
  fromDsp_status14/1 -> Terminator44/1
  fromDsp_status16/1 -> Terminator45/1
